simulink model "Equal"  (R2018a)
settings: Solver=VariableStepAuto  StartTime=0.0  StopTime=10.0  RelTol=1e-3
settings Model: Creator=midog  LastModifiedBy=midog

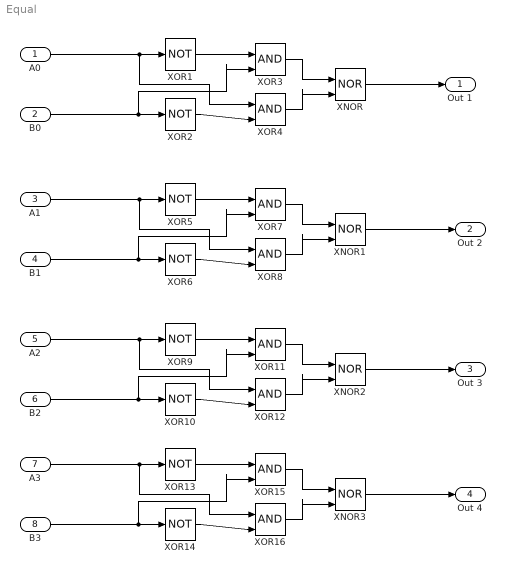
== system Equal ==
  A0 : Inport
  B0 : Inport  Port=2
  A1 : Inport  Port=3
  B1 : Inport  Port=4
  A2 : Inport  Port=5
  B2 : Inport  Port=6
  A3 : Inport  Port=7
  B3 : Inport  Port=8
  XNOR{,1..3} (4 alike) : Logic  Operator=NOR  IconShape=distinctive  AllPortsSameDT=off  OutDataTypeStr=boolean
  XOR{1..2,5..6,9..10,13..14} (8 alike) : Logic  Operator=NOT  IconShape=distinctive  AllPortsSameDT=off  OutDataTypeStr=boolean
  XOR{3..4,7..8,11..12,15..16} (8 alike) : Logic  IconShape=distinctive  AllPortsSameDT=off  OutDataTypeStr=boolean
  "Out 1 " : Outport
  Out 2 : Outport  Port=2
  Out 3 : Outport  Port=3
  Out 4 : Outport  Port=4
  wires:
  B0/1 -> XOR2/1, XOR3/2
  XOR1/1 -> XOR3/1
  XOR2/1 -> XOR4/2
  A0/1 -> XOR1/1, XOR4/1
  XOR4/1 -> XNOR/2
  XOR3/1 -> XNOR/1
  B1/1 -> XOR6/1, XOR7/2
  XOR8/1 -> XNOR1/2
  XOR6/1 -> XOR8/2
  XOR5/1 -> XOR7/1
  XOR7/1 -> XNOR1/1
  A1/1 -> XOR5/1, XOR8/1
  B2/1 -> XOR10/1, XOR11/2
  XOR12/1 -> XNOR2/2
  XOR10/1 -> XOR12/2
  XOR9/1 -> XOR11/1
  XOR11/1 -> XNOR2/1
  A2/1 -> XOR9/1, XOR12/1
  B3/1 -> XOR14/1, XOR15/2
  XOR16/1 -> XNOR3/2
  XOR14/1 -> XOR16/2
  XOR13/1 -> XOR15/1
  XOR15/1 -> XNOR3/1
  A3/1 -> XOR13/1, XOR16/1
  XNOR/1 -> "Out 1 "/1
  XNOR1/1 -> Out 2/1
  XNOR2/1 -> Out 3/1
  XNOR3/1 -> Out 4/1
